simulink model "Complete_Simulation"  (R2022b)
settings: Solver=ode5  StartTime=0.0  StopTime=2  FixedStep=1e-5  RelTol=1e-3
undefined symbols (not defined in the file or in its folder): conv
settings Model: Creator=gotta  LastModifiedBy=gotta
settings SolverCC: ZeroCrossAlgorithm=Adaptive
settings DebuggingCC: IgnoredZcDiagnostic=none
settings SimscapeCC: ExplicitSolverDiagnosticOptions=none

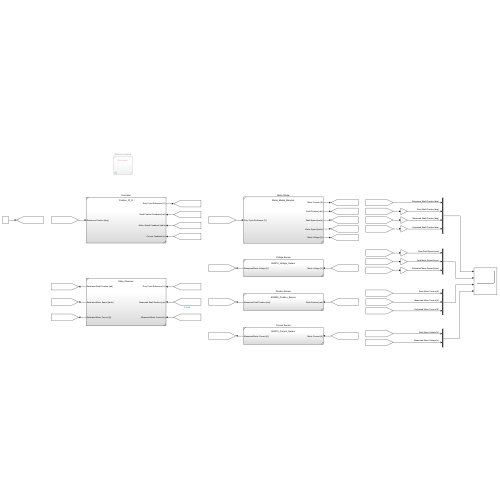
[thumbnail: Simulink's stored preview of the top-level diagram]
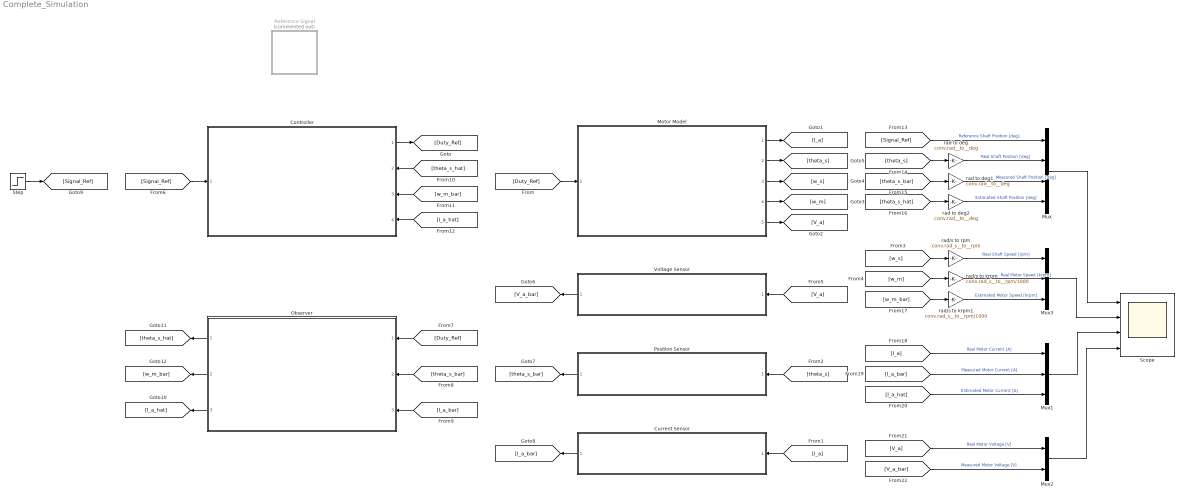
== system Complete_Simulation ==
  Controller : Subsystem  ReferencedSubsystem=Position_PI_D
      settings: PortSchema="{\"entries\":[{\"content\":{\"sides\":[{\"content\":{\"connectorIds\":[\"In1\"]},\"type\":\"ConnectorPlacement.EquallySpacedRectSide\",\"uuid\":\"0ebfbf0c-bc8e-4a80-a812-92a02abbf5a8\"},{\"content\":{\"connectorIds\":[\"Out1\",\"In2\",\"In3\",\"In4\"],\"side\":\"RIGHT\"},\"type\":\"ConnectorPlacement.EquallySpacedRectSide\",\"uuid\":\"6258934a-1c55-46d5-8b1d-537e4f4bfcdc\"},{\"content\":{\"connectorIds\":[],\"side\":\"TOP\"},\"type\":\"ConnectorPlacement.EquallySpacedRectSide\",\"uuid\":\"bd572b6a-f922-4437-a5b6-039a6e6ec46d\"}]},\"type\":\"ConnectorPlacement.EquallySpacedConnector\",\"uuid\":\"e83fe900-d361-4bcb-bab9-20465d904794\"}],\"packageUris\":[\"http://schema.mathworks.com/mf0/Connector/R2020b\"],\"version\":\"1.0\"}"
  Current Sensor : Subsystem  ReferencedSubsystem=INA219_Current_Sensor
  Motor Model : Subsystem  ReferencedSubsystem=Motor_Model_Simulink
  Mux : Mux
  Mux1 : Mux  Inputs=3
  Mux2 : Mux  Inputs=2
  Mux3 : Mux  Inputs=3
  Observer : Subsystem  ReferencedSubsystem=State_Observer
  Position Sensor : Subsystem  ReferencedSubsystem=AS5600_Position_Sensor
  Reference Signal : Subsystem  Commented=on  ReferencedSubsystem=<file name>
  Scope : Scope  NumInputPorts=4
  Step : Step  Time=0.2  After=180  SampleTime=0
  Voltage Sensor : Subsystem  ReferencedSubsystem=INA219_Voltage_Sensor
  rad to deg : Gain  Gain=conv.rad__to__deg
  rad to deg1 : Gain  Gain=conv.rad__to__deg
  rad to deg2 : Gain  Gain=conv.rad__to__deg
  rad/s to krpm : Gain  Gain=conv.rad_s__to__rpm/1000
  rad/s to krpm1 : Gain  Gain=conv.rad_s__to__rpm/1000
  rad/s to rpm : Gain  Gain=conv.rad_s__to__rpm
  wires:
  rad to deg/1 -> Mux/2  "Real Shaft Position [deg]"
  rad to deg1/1 -> Mux/3  "Measured Shaft Position [deg]"
  rad/s to krpm/1 -> Mux3/2  "Real Motor Speed [krpm]"
  rad/s to rpm/1 -> Mux3/1  "Real Shaft Speed [rpm]"
  rad/s to krpm1/1 -> Mux3/3  "Estimated Motor Speed [krpm]"
  Controller/1 -> [Duty_Ref]
  [Duty_Ref] -> Motor Model/1
  Motor Model/1 -> [I_a]
  Motor Model/2 -> [theta_s]
  Motor Model/5 -> [V_a]
  Motor Model/4 -> [w_m]
  Motor Model/3 -> [w_s]
  [V_a] -> Voltage Sensor/1
  [theta_s] -> Position Sensor/1
  [I_a] -> Current Sensor/1
  Current Sensor/1 -> [I_a_bar]
  Position Sensor/1 -> [theta_s_bar]
  Voltage Sensor/1 -> [V_a_bar]
  Step/1 -> [Signal_Ref]
  [Signal_Ref] -> Controller/1
  [I_a_bar] -> Observer/3
  Observer/1 -> [theta_s_hat]
  [theta_s_hat] -> Controller/2
  Observer/3 -> [I_a_hat]
  [I_a_hat] -> Controller/4
  Observer/2 -> [w_m_bar]
  [w_m_bar] -> Controller/3
  [Signal_Ref] -> Mux/1  "Reference Shaft Position [deg]"
  [theta_s] -> rad to deg/1
  [theta_s_bar] -> rad to deg1/1
  [theta_s_hat] -> rad to deg2/1
  rad to deg2/1 -> Mux/4  "Estimated Shaft Position [deg]"
  [w_m_bar] -> rad/s to krpm1/1
  [w_m] -> rad/s to krpm/1
  [w_s] -> rad/s to rpm/1
  [I_a] -> Mux1/1  "Real Motor Current [A]"
  [I_a_bar] -> Mux1/2  "Measured Motor Current [A]"
  [I_a_hat] -> Mux1/3  "Estimated Motor Current [A]"
  [V_a] -> Mux2/1  "Real Motor Voltage [V]"
  [V_a_bar] -> Mux2/2  "Measured Motor Voltage [V]"
  Mux/1 -> Scope/1
  Mux3/1 -> Scope/2
  Mux1/1 -> Scope/3
  Mux2/1 -> Scope/4
  [Duty_Ref] -> Observer/1
  [theta_s_bar] -> Observer/2

== system Complete_Simulation/Reference Signal ==
